simulink model "model31"  (R2022a)
settings: Solver=VariableStepAuto  StartTime=0.0  StopTime=10.0  RelTol=1e-3
values from neighbouring files (symbols this model uses):
  A = [   0    1 ... (first row only)    [config.m]    (also in task2.m = A + [0   0; task3.m = A + [0   0)
  A_m = [     0      1 ... (first row only)    [config.m]
  b = [0 ... (first row only)    [config.m]
  b_m = [0 ... (first row only)    [config.m]
  gamma = 100    [task3.m]
  k = b_0/a_m_0    (= 0.015552)    [config.m]
  P = lyap(A_m', Q)    [config.m]
  x_0 = [1; 0]    [config.m]
settings Model: Creator=Vvlad  LastModifiedBy=Vvlad

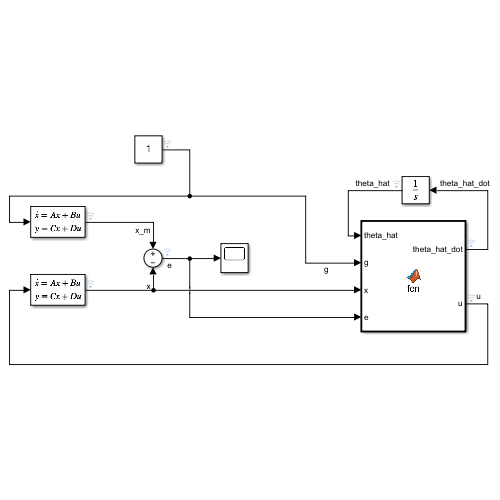
[thumbnail: Simulink's stored preview of the top-level diagram]
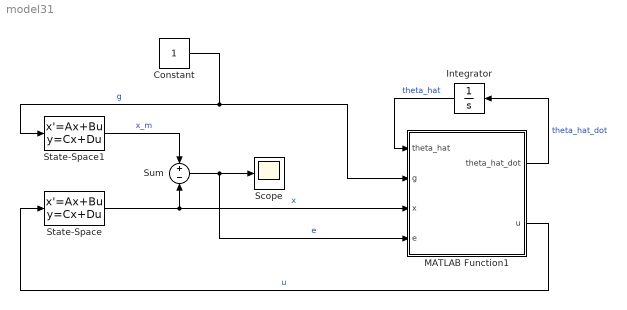
== system model31 ==
  Constant : Constant
  Integrator : Integrator
  MATLAB Function1 : MATLAB Function  TreatAsAtomicUnit=on
  Scope : Scope
  State-Space : StateSpace  A=A  B=b  C=eye(2)  D=[0;0]  InitialCondition=x_0
  State-Space1 : StateSpace  A=A_m  B=b_m  C=eye(2)  D=[0;0]  InitialCondition=0
  Sum : Sum  Inputs=+-
  wires:
  State-Space1/1 -> Sum/1  "x_m"
  State-Space/1 -> Sum/2, MATLAB Function1/3(x)  "x"
  Constant/1 -> State-Space1/1, MATLAB Function1/2(g)  "g"
  MATLAB Function1/2(u) -> State-Space/1  "u"
  Sum/1 -> MATLAB Function1/4(e), Scope/1  "e"
  MATLAB Function1/1(theta_hat_dot) -> Integrator/1  "theta_hat_dot"
  Integrator/1 -> MATLAB Function1/1(theta_hat)  "theta_hat"

== matlab function model31/MATLAB Function1 ==
  data: theta_hat input; theta_hat_dot output; g input; x input; e input; k parameter; P parameter; b parameter; u output; gamma parameter
function [theta_hat_dot, u]  = fcn(theta_hat, g, x, e, k, P, b, gamma)

u = theta_hat'*x + g/k;
theta_hat_dot = gamma*x*b'*P*e;
